simulink model "SolarPanel_Test"  (R2022a)
settings: Solver=VariableStepAuto  StartTime=0.0  StopTime=100.0  RelTol=1e-3  AbsTol=1e-3
libraries: nesl_utility x5, fl_lib x4, simulink x1
settings Model: Creator=michaelfsb  LastModifiedBy=michaelfsb
settings SolverCC: AutoScaleAbsTol=off  AlgebraicLoopSolver=TrustRegion  MaxZcPerStep=1
settings DebuggingCC: UnconnectedInputMsg=warning  UnconnectedOutputMsg=warning  UnconnectedLineMsg=warning  SymbolicDimsDataTypeCodeGenerationDiagnostic=none  SFMachineParentedDataDiag=warning
settings SFSimCC: CustomCodeUndefinedFunction=UseInterfaceOnly
settings RTWCC: DLArmComputeVersion=19.05
settings SimscapeCC: SimscapeLogType=all  SimscapeLogSimulationStatistics=on  SimscapeLogDataHistory=10000

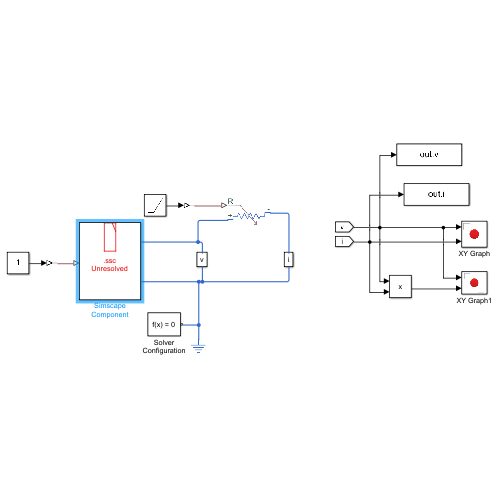
[thumbnail: Simulink's stored preview of the top-level diagram]
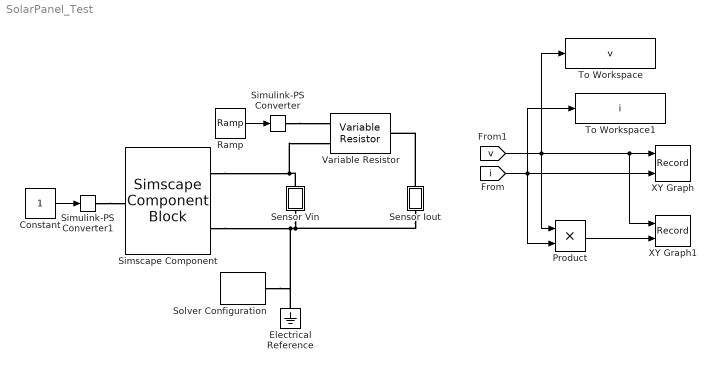
== system SolarPanel_Test ==
  Constant : Constant
  Electrical Reference : fl_lib/Electrical/Electrical Elements/Electrical Reference
      settings: SourceProductBaseCode=PW,SS,VE
  Product : Product
  Ramp : simulink/Sources/Ramp  slope=10  start=0  InitialOutput=0
  Sensor Vin : Subsystem
      mask Display: disp('v')
  Sensor Iout : Subsystem
      mask Display: disp('i')
  Simscape Component : SimscapeComponentBlock  SourceFile=SolarPanel  ComponentPath=SolarPanel  ComponentVariants="[\"SolarPanel\"]"  ComponentVariantNames="[\"SolarPanel\"]"  ClassName=SolarPanel  SchemaVersion=1  Nps=8  Nss=300  T=298.15 K  Tr=298.15 K  Isc=3.27 A  Kl=0.0017 A/K  Ior=2.0793e-6 A  Ego=1.1 V  A=1.6  i_specify=off  i_priority=None  i=0 A  i_nominal_specify=off  i_nominal_unit=A  i_nominal_value=1  v_specify=off  v_priority=None  v=0 V  v_nominal_specify=off  v_nominal_unit=V  v_nominal_value=1
      settings: CopyFcn=simscape.engine.sli.internal.componentblockcallback(gcbh,'COPY')  PreCopyFcn=simscape.engine.sli.internal.componentblockcallback(gcbh,'PRECOPY')  PreDeleteFcn=simscape.engine.sli.internal.componentblockcallback(gcbh,'PREDELETE')  InternalSimscapePortConfiguration="{\"Bottom\":[],\"Left\":[{\"id\":\"lambda\",\"label\":\"l\",\"type\":\"input\"}],\"Right\":[{\"id\":\"p\",\"label\":\"+\",\"type\":\"foundation.electrical.electrical\"},{\"id\":\"n\",\"label\":\"-\",\"type\":\"foundation.electrical.electrical\"}],\"Top\":[]}"
      mask Type: SolarPanel
  Simulink-PS Converter : nesl_utility/Simulink-PS Converter  PhysicalDomain=network_engine_domain  SubClassName=ps_input  LeftPortType=input  RightPortType=output  PseudoPeriodic=off  Frequencies=[]  NoiseDistribution=none  NoiseParameters=[]  Unit=1  AffineConversion=off  FilteringAndDerivatives=provide  SimscapeFilterOrder=1  InputFilterTimeConstant=0.001  UdotUserProvided=0
      settings: SourceProductBaseCode=SS,PW,VE
  Simulink-PS Converter1 : nesl_utility/Simulink-PS Converter  PhysicalDomain=network_engine_domain  SubClassName=ps_input  LeftPortType=input  RightPortType=output  PseudoPeriodic=off  Frequencies=[]  NoiseDistribution=none  NoiseParameters=[]  Unit=1  AffineConversion=off  FilteringAndDerivatives=provide  SimscapeFilterOrder=1  InputFilterTimeConstant=0.001  UdotUserProvided=0
      settings: SourceProductBaseCode=SS,PW,VE
  Solver Configuration : nesl_utility/Solver Configuration  PhysicalDomain=network_engine_domain  SubClassName=solver  LeftPortType=input  RightPortType=generic  Tones=[]  Harmonics=[]  SimulateNoise=off  Profile=off  UseLocalSampling=off  EnableSwitchedLinearOptims=on  FrequencyDomain=off  UseCCode=off  RelTol=0.001  AbsTol=1e-06  MinStep=1e-09  ToWorkspace=off  RevertToSquareIcSolve=off  NumHomotopyIterations=100  PhasorMode=off  PhasorModeNumHarmonics=1  IndexReductionMethod=DerivativeReplacement  DoDC=off  ResidualTolerance=1e-09  UseLocalSolver=off  LocalSolverChoice=NE_BACKWARD_EULER_ADVANCER  LocalSolverSampleTime=0.001  DoFixedCost=off  MaxNonlinIter=3  MaxModeIter=2  ComputeImpulses=off  ImpulseIterations=2  LinearAlgebra=auto  LinearAlgebraNumThread=0  EquationFormulation=NE_TIME_EF  DelaysMemoryBudget=1024  AutomaticFiltering=on  FilteringTimeConstant=0.001  PartitionStorageMethod=AS_NEEDED  PartitionMemoryBudget=1024  PartitionMethod=ROBUST
      settings: SourceProductBaseCode=SS,PW,VE
  To Workspace : ToWorkspace  VariableName=v  SaveFormat=Timeseries  SampleTime=-1
  To Workspace1 : ToWorkspace  VariableName=i  SaveFormat=Timeseries  SampleTime=-1
  Variable Resistor : fl_lib/Electrical/Electrical Elements/Variable Resistor  Rmin=0 Ohm  i_specify=off  i_priority=None  i=0 A  i_nominal_specify=off  i_nominal_unit=A  i_nominal_value=1  v_specify=off  v_priority=None  v=0 V  v_nominal_specify=off  v_nominal_unit=V  v_nominal_value=1
      settings: SourceProductBaseCode=PW,SS,VE
  XY Graph : Record  VariableName=recordout1  FileSettingsInternal="{\"entries\":[{\"content\":{\"excelSettings\":{\"content\":{},\"type\":\"Streamout.ExcelSettings\"}},\"type\":\"Streamout.FileSettingStorage\",\"uuid\":\"582aae9d-54d2-4ab5-94df-a6ed52113ea4\"}],\"packageUris\":[\"http://schema.mathworks.com/mf0/streamout_blocks/R2020a\"],\"version\":\"1.0\"}"  Layout=[1 1]  SignalsInternal="{\"entries\":[{\"content\":{\"signals\":[{\"content\":{\"blockPath\":[\"SolarPanel_Test/XY Graph\"],\"channel\":[],\"dimensions\":[1],\"domain\":\"SolarPanel_Test/XY Graph\",\"lineColor\":\"#a2142f\",\"plots\":[1],\"port\":1,\"sid\":[],\"signalID\":45,\"signalName\":\"From1\"},\"type\":\"RecordBlkView.Signal\",\"uuid\":\"1bd66ce5-be13-4120-9e52-90a4bc8aa342\"},{\"content\":{\"blockPath\":[\"SolarPanel_Test/XY Graph\"],\"channel\":[],\"dimensions\":[1],\"domain\":\"SolarPanel_Test/XY Graph\",\"lineColor\":\"#139fff\",\"plots\":[1],\"port\":2,\"sid\":[],\"signalID\":48,\"signalName\":\"From\"},\"type\":\"RecordBlkView.Signal\",\"uuid\":\"09c3b4d8-709c-4647-baff-7c66b46fa63e\"}]},\"type\":\"RecordBlkView.InputSignals\",\"uuid\":\"3f67fb1c-4a11-4742-8a9c-1677151b2618\"}],\"packageUris\":[\"http://schema.mathworks.com/mf0/streamout_blocks/R2020a\"],\"version\":\"1.0\"}"  VisualizationBindings="{\"xyplotplugin\":{\"info\":[{\"series\":[{\"bindingParametersList\":[{\"parameter\":\"X-Axis\",\"signalID\":45,\"signalName\":\"From1\"},{\"parameter\":\"Y-Axis\",\"signalID\":48,\"signalName\":\"From\"}],\"seriesID\":27191}],\"subplotID\":1}]}}"  CompatibilityTag=XY
  XY Graph1 : Record  VariableName=recordout2  RecordToWorkspace=on  FileSettingsInternal="{\"entries\":[{\"content\":{\"excelSettings\":{\"content\":{},\"type\":\"Streamout.ExcelSettings\"}},\"type\":\"Streamout.FileSettingStorage\",\"uuid\":\"4600882f-fa09-41a8-9769-2c2348c04620\"}],\"packageUris\":[\"http://schema.mathworks.com/mf0/streamout_blocks/R2020a\"],\"version\":\"1.0\"}"  Layout=[1 1]  SignalsInternal="{\"entries\":[{\"content\":{\"signals\":[{\"content\":{\"blockPath\":[\"SolarPanel_Test/XY Graph1\"],\"channel\":[],\"dimensions\":[1],\"domain\":\"SolarPanel_Test/XY Graph1\",\"lineColor\":\"#a2142f\",\"plots\":[1],\"port\":1,\"sid\":[],\"signalID\":53,\"signalName\":\"From1\"},\"type\":\"RecordBlkView.Signal\",\"uuid\":\"c869dff5-5728-4b35-a8b8-79c431233664\"},{\"content\":{\"blockPath\":[\"SolarPanel_Test/XY Graph1\"],\"channel\":[],\"dimensions\":[1],\"domain\":\"SolarPanel_Test/XY Graph1\",\"lineColor\":\"#139fff\",\"plots\":[1],\"port\":2,\"sid\":[],\"signalID\":56,\"signalName\":\"Product\"},\"type\":\"RecordBlkView.Signal\",\"uuid\":\"77bcd8d5-a155-4a40-a525-2ae4ed209140\"}]},\"type\":\"RecordBlkView.InputSignals\",\"uuid\":\"bd4e724a-be84-4660-8a4e-0ad8b7be6afa\"}],\"packageUris\":[\"http://schema.mathworks.com/mf0/streamout_blocks/R2020a\"],\"version\":\"1.0\"}"  VisualizationBindings="{\"xyplotplugin\":{\"info\":[{\"series\":[{\"bindingParametersList\":[{\"parameter\":\"X-Axis\",\"signalID\":53,\"signalName\":\"From1\"},{\"parameter\":\"Y-Axis\",\"signalID\":56,\"signalName\":\"Product\"}],\"seriesID\":17585}],\"subplotID\":1}]}}"  CompatibilityTag=XY
  wires:
  Constant/1 -> Simulink-PS Converter1/1
  Ramp/1 -> Simulink-PS Converter/1
  [v] -> To Workspace/1, XY Graph1/1, XY Graph/1, Product/1
  [i] -> To Workspace1/1, XY Graph/2, Product/2
  Product/1 -> XY Graph1/2
  connections:
  Simulink-PS Converter/RConn1 -- Variable Resistor/LConn1
  Simscape Component/RConn1 -- Sensor Vin/RConn1 -- Variable Resistor/LConn2
  Sensor Iout/RConn1 -- Variable Resistor/RConn1
  Sensor Vin/LConn1 -- Sensor Iout/LConn1 -- Electrical Reference/LConn1 -- Solver Configuration/RConn1 -- Simscape Component/RConn2
  Simulink-PS Converter1/RConn1 -- Simscape Component/LConn1

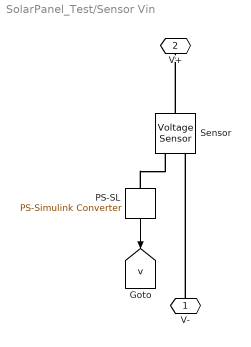
== system SolarPanel_Test/Sensor Vin ==
  PS-SL : nesl_utility/PS-Simulink Converter  PhysicalDomain=network_engine_domain  SubClassName=ps_output  LeftPortType=input  RightPortType=output  PseudoPeriodic=off  Frequencies=[]  VectorFormat=1-D array  Unit=1  AffineConversion=off
      settings: SourceProductBaseCode=SS,PW,VE
  Sensor : fl_lib/Electrical/Electrical Sensors/Voltage Sensor
      settings: SourceProductBaseCode=PW,SS,VE
  V- : PMIOPort  Side=Left
  V+ : PMIOPort  Port=2  Side=Right
  tag scope: v=global
  wires:
  PS-SL/1 -> [v]
  connections:
  PS-SL/LConn1 -- Sensor/RConn1
  Sensor/LConn1 -- V+/RConn1
  V-/RConn1 -- Sensor/RConn2

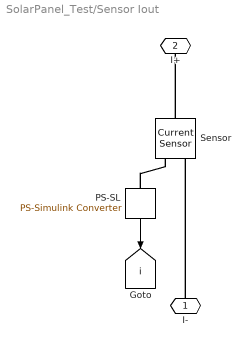
== system SolarPanel_Test/Sensor Iout ==
  PS-SL : nesl_utility/PS-Simulink Converter  PhysicalDomain=network_engine_domain  SubClassName=ps_output  LeftPortType=input  RightPortType=output  PseudoPeriodic=off  Frequencies=[]  VectorFormat=1-D array  Unit=1  AffineConversion=off
      settings: SourceProductBaseCode=SS,PW,VE
  Sensor : fl_lib/Electrical/Electrical Sensors/Current Sensor
      settings: SourceProductBaseCode=PW,SS,VE
  I- : PMIOPort  Side=Left
  I+ : PMIOPort  Port=2  Side=Right
  tag scope: i=global
  wires:
  PS-SL/1 -> [i]
  connections:
  PS-SL/LConn1 -- Sensor/RConn1
  Sensor/LConn1 -- I+/RConn1
  I-/RConn1 -- Sensor/RConn2
